simulink library "ESTS_FRIC_HILO_STATE"  (R2024b)
settings: Solver=VariableStepAuto  StartTime=0.0  StopTime=10.0  RelTol=1e-3
undefined symbols (not defined in the file or in its folder): ESTS_c_TiSample_s, ESTS_FRIC_HILO_STATE_p_TiDbnChart_s, ESTS_p_SwtHiMue_na
settings Model: Creator=blatak  LastModifiedBy=blatak

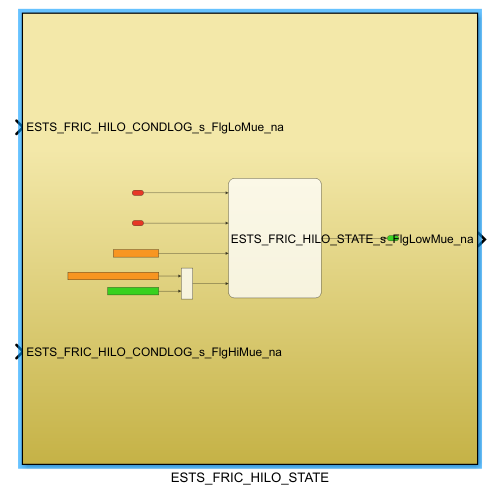
[thumbnail: Simulink's stored preview of the top-level diagram]
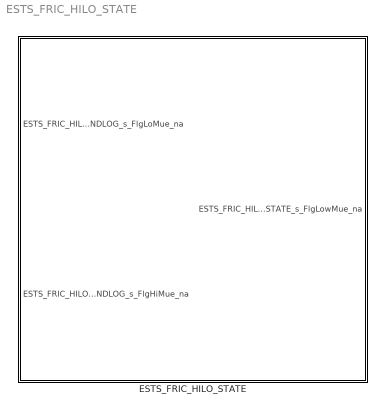
== system ESTS_FRIC_HILO_STATE ==
  ESTS_FRIC_HILO_STATE : Subsystem

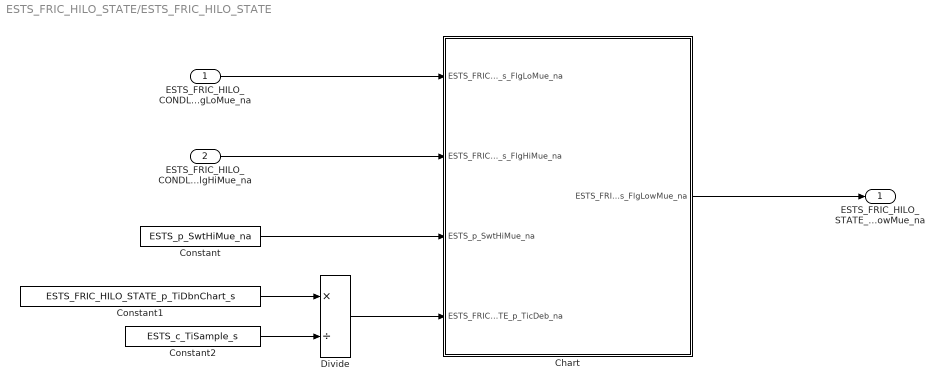
== system ESTS_FRIC_HILO_STATE/ESTS_FRIC_HILO_STATE ==
  ESTS_FRIC_HILO_CONDLOG_s_FlgLoMue_na : Inport
  ESTS_FRIC_HILO_CONDLOG_s_FlgHiMue_na : Inport  Port=2
  Chart : Stateflow chart  TreatAsAtomicUnit=on
  Constant : Constant  Value=ESTS_p_SwtHiMue_na
  Constant1 : Constant  Value=ESTS_FRIC_HILO_STATE_p_TiDbnChart_s
  Constant2 : Constant  Value=ESTS_c_TiSample_s
  Divide : Product  Inputs=*/
  ESTS_FRIC_HILO_STATE_s_FlgLowMue_na : Outport
  wires:
  Divide/1 -> Chart/4(ESTS_FRIC_HILO_STATE_p_TicDeb_na)
  Constant/1 -> Chart/3(ESTS_p_SwtHiMue_na)
  ESTS_FRIC_HILO_CONDLOG_s_FlgLoMue_na/1 -> Chart/1(ESTS_FRIC_HILO_CONDLOG_s_FlgLoMue_na)
  Constant1/1 -> Divide/1
  ESTS_FRIC_HILO_CONDLOG_s_FlgHiMue_na/1 -> Chart/2(ESTS_FRIC_HILO_CONDLOG_s_FlgHiMue_na)
  Chart/1(ESTS_FRIC_HILO_STATE_s_FlgLowMue_na) -> ESTS_FRIC_HILO_STATE_s_FlgLowMue_na/1
  Constant2/1 -> Divide/2

== stateflow chart ESTS_FRIC_HILO_STATE/Chart ==
  state HiMue
  state Possibly_low
  state Possibly_high
  state LoMue
  (default) -> (junction 6)
  (junction 6) -> (junction 14) [order 2]
  (junction 6) -> HiMue [order 1] : [ESTS_p_SwtHiMue_na]
      | {ESTS_FRIC_HILO_STATE_s_FlgLowMue_na=false;}
  (junction 14) -> (junction 17)
  (junction 26) -> HiMue
  (junction 25) -> (junction 26)
  HiMue -> Possibly_low : [ESTS_FRIC_HILO_CONDLOG_s_FlgLoMue_na]
  Possibly_high -> HiMue [order 1] : [after(ESTS_FRIC_HILO_STATE_p_TicDeb_na,tick)]
      | {ESTS_FRIC_HILO_STATE_s_FlgLowMue_na=false;}
  Possibly_high -> (junction 17) [order 2] : [ESTS_FRIC_HILO_CONDLOG_s_FlgLoMue_na]
  Possibly_low -> (junction 25) [order 2] : [ESTS_FRIC_HILO_CONDLOG_s_FlgHiMue_na]
  (junction 17) -> (junction 16)
  Possibly_low -> LoMue [order 1] : [after(ESTS_FRIC_HILO_STATE_p_TicDeb_na,tick)]
      | {ESTS_FRIC_HILO_STATE_s_FlgLowMue_na=true;}
  LoMue -> Possibly_high : [ESTS_FRIC_HILO_CONDLOG_s_FlgHiMue_na]
  (junction 16) -> LoMue : {ESTS_FRIC_HILO_STATE_s_FlgLowMue_na=true;}
  data: ESTS_FRIC_HILO_CONDLOG_s_FlgLoMue_na input; ESTS_FRIC_HILO_CONDLOG_s_FlgHiMue_na input; ESTS_p_SwtHiMue_na input; ESTS_FRIC_HILO_STATE_p_TicDeb_na input; ESTS_FRIC_HILO_STATE_s_FlgLowMue_na output
